simulink model "E1_3"  (R2021a)
settings: Solver=VariableStepAuto  StartTime=0.0  StopTime=100  RelTol=1e-3
settings Model: Creator=erlen  LastModifiedBy=erlen

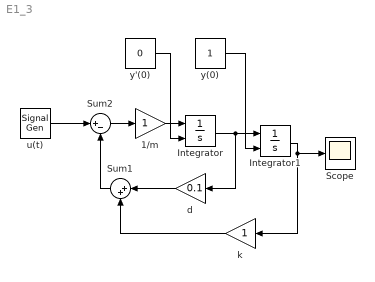
== system E1_3 ==
  1/m : Gain
  Integrator : Integrator  InitialConditionSource=external
  Integrator1 : Integrator  InitialConditionSource=external
  Scope : Scope
  Sum1 : Sum  Inputs=|++
  Sum2 : Sum  Inputs=|+-
  d : Gain  Gain=0.1
  k : Gain
  u(t) : SignalGenerator  Frequency=1/6.5
  y'(0) : Constant  Value=0
  y(0) : Constant
  wires:
  Integrator/1 -> Integrator1/1, d/1
  1/m/1 -> Integrator/1
  Integrator1/1 -> k/1, Scope/1
  Sum2/1 -> 1/m/1
  Sum1/1 -> Sum2/2
  u(t)/1 -> Sum2/1
  y'(0)/1 -> Integrator/2
  y(0)/1 -> Integrator1/2
  d/1 -> Sum1/1
  k/1 -> Sum1/2
